simulink model "band_3"  (Simulink 7.8)
settings: Solver=ode45  StartTime=0.0  StopTime=2  RelTol=1e-3
libraries: dsparch4 x10, dspsigops x8, dspsrcs4 x1
settings Model: Creator=svenhoffmann  LastModifiedBy=josef  ExtModeAutoUpdateStatusClock=off
settings DataIOCC: SignalLoggingName=sigsOut
settings OptimizationCC: InitFltsAndDblsToZero=on
settings DebuggingCC: SaveWithParameterizedLinksMsg=none  SignalResolutionControl=TryResolveAllWithWarning  SolverPrmCheckMsg=none  MultiTaskDSMMsg=warning  MultiTaskCondExecSysMsg=none  FcnCallInpInsideContextMsg=Use local settings  StrictBusMsg=None
settings HardwareCC: TargetUnknown=on
settings RTWCC: IncludeERTFirstTime=on
settings GRTTargetCC: TargetFcnLib=ansi_tfl_tmw.mat

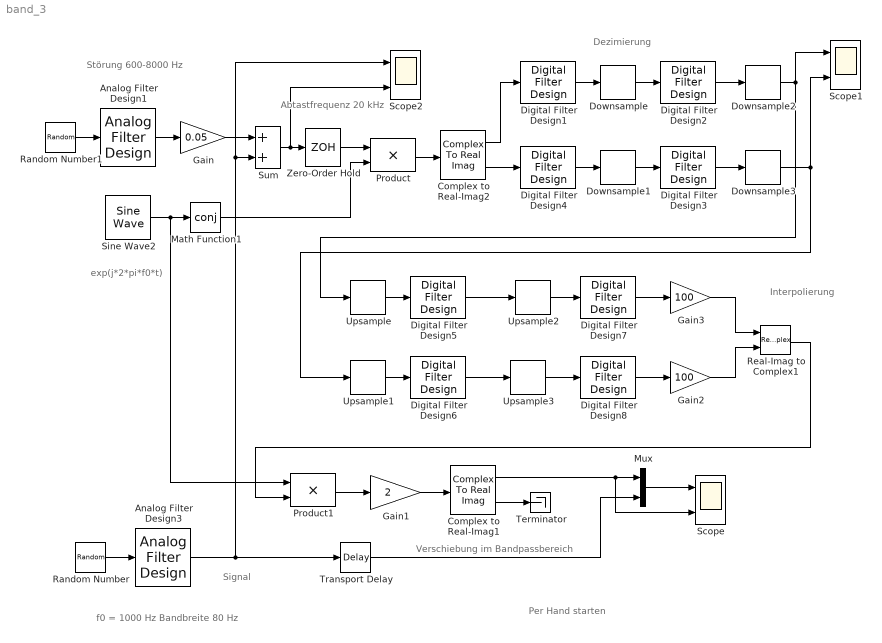
== system band_3 ==
  note: Signal
  note: exp(j*2*pi*f0*t)
  note: Störung
      | 600-8000 Hz
  note: f0 = 1000 Hz
      | Bandbreite
      | 80 Hz
  note: Abtastfrequenz
      | 20 kHz
  note: Dezimierung
  note: Interpolierung
  note: Verschiebung im Bandpassbereich
  note: Per Hand starten
  Analog Filter Design1 : dsparch4/Analog Filter Design  method=Chebyshev I  filttype=Bandpass  N=8  Wlo=2*pi*600  Whi=2*pi*8000  Rp=2  Rs=40
  Analog Filter Design3 : dsparch4/Analog Filter Design  method=Butterworth  filttype=Bandpass  N=8  Wlo=2*pi*960  Whi=2*pi*1040  Rp=2  Rs=40
  Complex to Real-Imag1 : ComplexToRealImag
  Complex to Real-Imag2 : ComplexToRealImag
  Digital Filter Design{1..8} (8 alike) : dsparch4/Digital Filter Design  mwdsp_browser_bugfix_var=off
  Downsample{,1..3} (4 alike) : dspsigops/Downsample  N=10  phase=0  InputProcessing=Inherited (this choice will be removed - see release notes)  RateOptions=Enforce single-rate processing  smode=Allow multirate  fmode=Maintain input frame size  ic=0
  Gain : Gain  Gain=0.05  SaturateOnIntegerOverflow=on  OutDataTypeStr=Inherit: Same as input  ParamDataTypeStr=Inherit: Same as input
  Gain1 : Gain  Gain=2  SaturateOnIntegerOverflow=on  OutDataTypeStr=Inherit: Same as input  ParamDataTypeStr=Inherit: Same as input
  Gain2 : Gain  Gain=100  SaturateOnIntegerOverflow=on  OutDataTypeStr=Inherit: Same as input  ParamDataTypeStr=Inherit: Same as input
  Gain3 : Gain  Gain=100  SaturateOnIntegerOverflow=on  OutDataTypeStr=Inherit: Same as input  ParamDataTypeStr=Inherit: Same as input
  Math Function1 : Math  Operator=conj  SaturateOnIntegerOverflow=on
  Mux : Mux  Inputs=2
  Product : Product  SaturateOnIntegerOverflow=on  OutDataTypeStr=Inherit: Same as first input
  Product1 : Product  SaturateOnIntegerOverflow=on  OutDataTypeStr=Inherit: Same as first input
  Random Number : RandomNumber  SampleTime=0
  Random Number1 : RandomNumber  SampleTime=0
  Real-Imag to Complex1 : RealImagToComplex
  Scope : Scope  NumInputPorts=2
      settings: YMin=-0.15~-0.15  YMax=0.15~0.15  MaxDataPoints=500000
  Scope1 : Scope  NumInputPorts=2
      settings: YMin=-0.06~-0.05  YMax=0.05~0.07  MaxDataPoints=500000
  Scope2 : Scope  NumInputPorts=2
      settings: YMin=-0.15~-0.2  YMax=0.15~0.2  SaveName=ScopeData2  MaxDataPoints=500000
  Sine Wave2 : dspsrcs4/Sine Wave  Amplitude=1  Frequency=1000  Phase=0  SampleMode=Discrete  OutComplex=Complex  CompMethod=Table lookup  TableSize=Speed  SampleTime=1/20000  SamplesPerFrame=1  ResetState=Restart at time zero  dataType=double  wordLen=16  udDataType=sfix(16)  fracBitsMode=Best precision  numFracBits=15  OutDataTypeStr=double  LastOutDataTypeStr=double
      settings: additionalParams=on
  Sum : Sum  SaturateOnIntegerOverflow=on
  Terminator : Terminator
  Transport Delay : TransportDelay  DelayTime=60e-3  BufferSize=4096
  Upsample{,1..3} (4 alike) : dspsigops/Upsample  N=10  phase=0  InputProcessing=Inherited (this choice will be removed - see release notes)  RateOptions=Allow multirate processing  ic=0  mode=Unused parameter value
  Zero-Order Hold : ZeroOrderHold  SampleTime=1/20000
  wires:
  Random Number1/1 -> Analog Filter Design1/1
  Analog Filter Design1/1 -> Gain/1
  Gain/1 -> Sum/1
  Sum/1 -> Zero-Order Hold/1, Scope2/2
  Zero-Order Hold/1 -> Product/1
  Sine Wave2/1 -> Math Function1/1, Product1/1
  Mux/1 -> Scope/1
  Transport Delay/1 -> Mux/2
  Product1/1 -> Gain1/1
  Gain1/1 -> Complex to Real-Imag1/1
  Product/1 -> Complex to Real-Imag2/1
  Complex to Real-Imag2/1 -> Digital Filter Design1/1
  Complex to Real-Imag2/2 -> Digital Filter Design4/1
  Digital Filter Design1/1 -> Downsample/1
  Digital Filter Design4/1 -> Downsample1/1
  Real-Imag to Complex1/1 -> Product1/2
  Math Function1/1 -> Product/2
  Random Number/1 -> Analog Filter Design3/1
  Downsample/1 -> Digital Filter Design2/1
  Downsample1/1 -> Digital Filter Design3/1
  Upsample/1 -> Digital Filter Design5/1
  Upsample1/1 -> Digital Filter Design6/1
  Digital Filter Design6/1 -> Upsample3/1
  Complex to Real-Imag1/1 -> Mux/1, Scope/2
  Analog Filter Design3/1 -> Transport Delay/1, Sum/2, Scope2/1
  Gain3/1 -> Real-Imag to Complex1/1
  Gain2/1 -> Real-Imag to Complex1/2
  Digital Filter Design2/1 -> Downsample2/1
  Downsample2/1 -> Scope1/1, Upsample/1
  Digital Filter Design3/1 -> Downsample3/1
  Downsample3/1 -> Scope1/2, Upsample1/1
  Upsample2/1 -> Digital Filter Design7/1
  Digital Filter Design5/1 -> Upsample2/1
  Digital Filter Design7/1 -> Gain3/1
  Upsample3/1 -> Digital Filter Design8/1
  Digital Filter Design8/1 -> Gain2/1
  Complex to Real-Imag1/2 -> Terminator/1
